simulink model "SF105A_MotCurrRegVltgLimr"  (R2013b)
settings: Solver=FixedStepDiscrete  SolverMode=SingleTasking  StartTime=0.0  StopTime=1  FixedStep=0.00025  RelTol=1e-3
undefined symbols (not defined in the file): ARCHGLBPRM_2OVERSQRT3_ULS_F32, ARCHGLBPRM_2PI_ULS_F32, BRDGVLTGHILIM_VOLT_F32, ELECGLBPRM_PWMPERDNOMX2_SEC_F32, F32TOU16OVR2PI_ULS_F32, MotCurrRegCfgCurrLoopSecOrderTrfFctEna, MotCurrRegCfgMotRVirtDax, MotCurrRegCfgMotRVirtQax, MotCurrRegVltgLimrCurrLoaScarSlewRate, MotCurrRegVltgLimrDaxAntiWdupCoeff, MotCurrRegVltgLimrDualEcuLoaScarSlewRate, MotCurrRegVltgLimrIvtrLoaScarSlewRate, MotCurrRegVltgLimrMotCurrPredEna, MotCurrRegVltgLimrMotCurrPredTi, MotCurrRegVltgLimrMotCurrQaxRefMdfnRplEna, MotCurrRegVltgLimrMotVltgBrdgFilEna, MotCurrRegVltgLimrMotVltgDaxIntglHiLim, MotCurrRegVltgLimrMotVltgDaxIntglLoLim, MotCurrRegVltgLimrMotVltgQaxFfFilEna, MotCurrRegVltgLimrMotVltgQaxIntglHiLim, MotCurrRegVltgLimrMotVltgQaxIntglLoLim, MotCurrRegVltgLimrQaxAntiWdupCoeff, MotCurrRegVltgLimrQaxAntiWdupScagDi, MotRefMdlFbCtrlDi, MotRefMdlIvtrDeadTiBrdgVltgSca, SysSt1, ZERO_VOLT_F32
libraries: NxtrLim x15, Fil x4, simulink x3, NxtrMax x2, NxtrMin x2
(part 4 of 5)

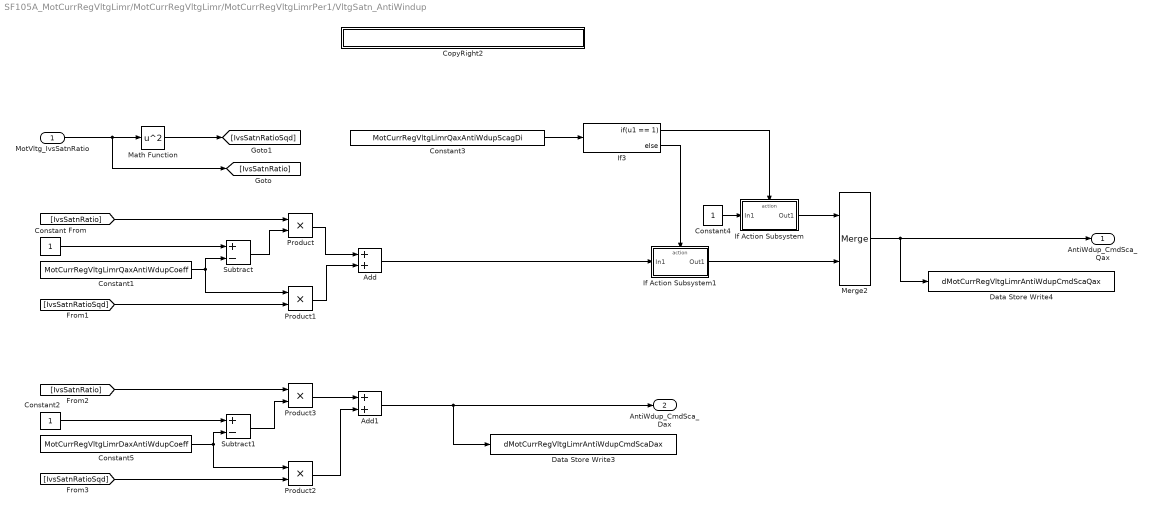
== system SF105A_MotCurrRegVltgLimr/MotCurrRegVltgLimr/MotCurrRegVltgLimrPer1/VltgSatn_AntiWindup ==
  MotVltg_IvsSatnRatio : Inport  RequirementInfo="{'linktype_rmi_doors' '0000bb44 (/E-STEER Core/SubSystem Specifications/Application Functions/SF99/SF105A Current Regulator and Voltage Limiter)' '#SF105A_130' 'true' 'REQ:  SF105A_130' '' ; 'linktype_rmi_doors' '0000bb44 (/E-STEER Core/SubSystem Specifications/Application Functions/SF99/SF105A Current Regulator and Voltage Limiter)' '#SF105A_130' 'true' 'REQ:  SF105A_130' '' } %GIDa_888bca64_0823_4deb_ba1d_307ad11fc636"
  Add : Sum  RequirementInfo="{'linktype_rmi_doors' '0000bb44 (/E-STEER Core/SubSystem Specifications/Application Functions/SF99/SF105A Current Regulator and Voltage Limiter)' '#SF105A_126' 'true' 'REQ:  SF105A_126' '' } %GIDa_812b0983_0c53_4cfa_9a51_643dbc79a070"
  Add1 : Sum  RequirementInfo="{'linktype_rmi_doors' '0000bb44 (/E-STEER Core/SubSystem Specifications/Application Functions/SF99/SF105A Current Regulator and Voltage Limiter)' '#SF105A_130' 'true' 'REQ:  SF105A_130' '' } %GIDa_2674bb96_c0b6_4cdb_b829_01729431041f"
  Constant : Constant  RequirementInfo="{'linktype_rmi_doors' '0000bb44 (/E-STEER Core/SubSystem Specifications/Application Functions/SF99/SF105A Current Regulator and Voltage Limiter)' '#SF105A_126' 'true' 'REQ:  SF105A_126' '' } %GIDa_a4ea031f_79fb_49ac_9d61_2a336d42d170"  OutDataTypeStr=single
  Constant1 : Constant  RequirementInfo="{'linktype_rmi_doors' '0000bb44 (/E-STEER Core/SubSystem Specifications/Application Functions/SF99/SF105A Current Regulator and Voltage Limiter)' '#SF105A_126' 'true' 'REQ:  SF105A_126' '' ; 'linktype_rmi_doors' '0000bb44 (/E-STEER Core/SubSystem Specifications/Application Functions/SF99/SF105A Current Regulator and Voltage Limiter)' '#SF105A_126' 'true' 'REQ:  SF105A_126' '' } %GIDa_f0528501_6455_46bb_9be1_873b38c0945c"  Value=MotCurrRegVltgLimrQaxAntiWdupCoeff
  Constant2 : Constant  RequirementInfo="{'linktype_rmi_doors' '0000bb44 (/E-STEER Core/SubSystem Specifications/Application Functions/SF99/SF105A Current Regulator and Voltage Limiter)' '#SF105A_130' 'true' 'REQ:  SF105A_130' '' } %GIDa_f1e0f24a_4abc_445f_8df3_e7d8a5290d26"  OutDataTypeStr=single
  Constant3 : Constant  RequirementInfo="{'linktype_rmi_doors' '0000bb44 (/E-STEER Core/SubSystem Specifications/Application Functions/SF99/SF105A Current Regulator and Voltage Limiter)' '#SF105A_126' 'true' 'REQ:  SF105A_126' '' } %GIDa_0a590627_be14_4a36_8e32_6ad02ffe62c3"  Value=MotCurrRegVltgLimrQaxAntiWdupScagDi
  Constant4 : Constant  RequirementInfo="{'linktype_rmi_doors' '0000bb44 (/E-STEER Core/SubSystem Specifications/Application Functions/SF99/SF105A Current Regulator and Voltage Limiter)' '#SF105A_126' 'true' 'REQ:  SF105A_126' '' } %GIDa_b2b2de9c_8926_4bf3_ad2c_18100fed640c"  OutDataTypeStr=single
  Constant5 : Constant  RequirementInfo="{'linktype_rmi_doors' '0000bb44 (/E-STEER Core/SubSystem Specifications/Application Functions/SF99/SF105A Current Regulator and Voltage Limiter)' '#SF105A_126' 'true' 'REQ:  SF105A_126' '' ; 'linktype_rmi_doors' '0000bb44 (/E-STEER Core/SubSystem Specifications/Application Functions/SF99/SF105A Current Regulator and Voltage Limiter)' '#SF105A_130' 'true' 'REQ:  SF105A_130' '' } %GIDa_6fe1152d_0e16_4530_a23a_94ed2f7f620d"  Value=MotCurrRegVltgLimrDaxAntiWdupCoeff
  CopyRight2 : Subsystem  Description=|  mask(Copyright Information){none=on}
      | Copyright info block.                                               
      |                                                                     
      | Place copyright information at the top of every subsystem in design.
      mask prompts: none "No parameters"
      mask help: Place copyright information at the top of every subsystem in design.
      mask Display:
      | NxtrConf = 'Nexteer Confidential';
      | 
      | sys = bdroot; %handle for the current model ("system")
      | first = get_param(sys,'Created');
      | if(isempty(first))
      |     first = datestr(now,'yyyy');
      | else
      |     first = first(end-3:end);  %year is last four digits
      | end
      | 
      | last = get_param(sys,'LastModifiedDate');
      | if isempty(last)
      |     last = datestr(now,'yyyy');
      | else
      |     last = last(end-3:end);
      | end
      | 
      | if strcmp(first,last)
      |     fprintf('%s -- Copyright %s Nexteer',NxtrConf,first)
      | else
      |     fprintf('%s -- %s%s- %s Nexteer',NxtrConf,char(169),first,last)
      | end
  Data Store Write3 : DataStoreWrite  RequirementInfo="{'linktype_rmi_doors' '0000bb44 (/E-STEER Core/SubSystem Specifications/Application Functions/SF99/SF105A Current Regulator and Voltage Limiter)' '#SF105A_141' 'true' 'REQ:  SF105A_141' '' } %GIDa_d69d978d_8d8c_4eb5_8eb7_5cf010971c8b"  DataStoreName=dMotCurrRegVltgLimrAntiWdupCmdScaDax
  Data Store Write4 : DataStoreWrite  RequirementInfo="{'linktype_rmi_doors' '0000bb44 (/E-STEER Core/SubSystem Specifications/Application Functions/SF99/SF105A Current Regulator and Voltage Limiter)' '#SF105A_141' 'true' 'REQ:  SF105A_141' '' } %GIDa_9849020c_0cb1_40e6_a462_20415501e4e7"  DataStoreName=dMotCurrRegVltgLimrAntiWdupCmdScaQax
  If Action Subsystem : Subsystem  RequirementInfo="{'linktype_rmi_doors' '0000bb44 (/E-STEER Core/SubSystem Specifications/Application Functions/SF99/SF105A Current Regulator and Voltage Limiter)' '#SF105A_126' 'true' 'REQ:  SF105A_126' '' } %GIDa_c49f3131_c39a_4483_bd39_15998722cd10"  TreatAsAtomicUnit=on
  If Action Subsystem1 : Subsystem  RequirementInfo="{'linktype_rmi_doors' '0000bb44 (/E-STEER Core/SubSystem Specifications/Application Functions/SF99/SF105A Current Regulator and Voltage Limiter)' '#SF105A_126' 'true' 'REQ:  SF105A_126' '' } %GIDa_0be6e736_8039_4cb8_9da1_1d96e36153a9"  TreatAsAtomicUnit=on
  If3 : If  RequirementInfo="{'linktype_rmi_doors' '0000bb44 (/E-STEER Core/SubSystem Specifications/Application Functions/SF99/SF105A Current Regulator and Voltage Limiter)' '#SF105A_126' 'true' 'REQ:  SF105A_126' '' } %GIDa_dbf56d85_10ab_48c7_a6a3_82cb7cfa18de"  IfExpression=u1 == 1
  Math Function : Math  RequirementInfo="{'linktype_rmi_doors' '0000bb44 (/E-STEER Core/SubSystem Specifications/Application Functions/SF99/SF105A Current Regulator and Voltage Limiter)' '#SF105A_130' 'true' 'REQ:  SF105A_130' '' ; 'linktype_rmi_doors' '0000bb44 (/E-STEER Core/SubSystem Specifications/Application Functions/SF99/SF105A Current Regulator and Voltage Limiter)' '#SF105A_130' 'true' 'REQ:  SF105A_130' '' } %GIDa_b09f1dfa_1331_43ca_8f8b_9feb85653759"  Operator=square  SaturateOnIntegerOverflow=on
  Merge2 : Merge  RequirementInfo="{'linktype_rmi_doors' '0000bb44 (/E-STEER Core/SubSystem Specifications/Application Functions/SF99/SF105A Current Regulator and Voltage Limiter)' '#SF105A_126' 'true' 'REQ:  SF105A_126' '' } %GIDa_8d5f9f4e_85d5_4273_905f_4ef98e59c94a"
  Product : Product  RequirementInfo="{'linktype_rmi_doors' '0000bb44 (/E-STEER Core/SubSystem Specifications/Application Functions/SF99/SF105A Current Regulator and Voltage Limiter)' '#SF105A_126' 'true' 'REQ:  SF105A_126' '' } %GIDa_ea6027c8_8a1b_4f13_be09_e5e1cad10d1f"
  Product1 : Product  RequirementInfo="{'linktype_rmi_doors' '0000bb44 (/E-STEER Core/SubSystem Specifications/Application Functions/SF99/SF105A Current Regulator and Voltage Limiter)' '#SF105A_126' 'true' 'REQ:  SF105A_126' '' } %GIDa_f8ee43f2_9342_474e_acda_6fc019895fb8"
  Product2 : Product  RequirementInfo="{'linktype_rmi_doors' '0000bb44 (/E-STEER Core/SubSystem Specifications/Application Functions/SF99/SF105A Current Regulator and Voltage Limiter)' '#SF105A_130' 'true' 'REQ:  SF105A_130' '' } %GIDa_1c2ad4c0_5990_4d45_bbe5_57d9582fe383"
  Product3 : Product  RequirementInfo="{'linktype_rmi_doors' '0000bb44 (/E-STEER Core/SubSystem Specifications/Application Functions/SF99/SF105A Current Regulator and Voltage Limiter)' '#SF105A_130' 'true' 'REQ:  SF105A_130' '' } %GIDa_0fc5ec00_cbe3_4725_98f5_b8cec8d7b237"
  Subtract : Sum  RequirementInfo="{'linktype_rmi_doors' '0000bb44 (/E-STEER Core/SubSystem Specifications/Application Functions/SF99/SF105A Current Regulator and Voltage Limiter)' '#SF105A_126' 'true' 'REQ:  SF105A_126' '' } %GIDa_ed1d9f08_fe01_45f1_add5_02a80c037d9d"  Inputs=+-
  Subtract1 : Sum  RequirementInfo="{'linktype_rmi_doors' '0000bb44 (/E-STEER Core/SubSystem Specifications/Application Functions/SF99/SF105A Current Regulator and Voltage Limiter)' '#SF105A_130' 'true' 'REQ:  SF105A_130' '' } %GIDa_badc02ff_cfe5_4c0b_9d95_39b5b5fe7a5f"  Inputs=+-
  AntiWdup_CmdSca_Qax : Outport  RequirementInfo="{'linktype_rmi_doors' '0000bb44 (/E-STEER Core/SubSystem Specifications/Application Functions/SF99/SF105A Current Regulator and Voltage Limiter)' '#SF105A_126' 'true' 'REQ:  SF105A_126' '' } %GIDa_d17ed289_17c6_4f50_a1dc_ba7a5b94eaaa"
  AntiWdup_CmdSca_Dax : Outport  RequirementInfo="{'linktype_rmi_doors' '0000bb44 (/E-STEER Core/SubSystem Specifications/Application Functions/SF99/SF105A Current Regulator and Voltage Limiter)' '#SF105A_130' 'true' 'REQ:  SF105A_130' '' } %GIDa_6b63b34d_3c6d_43f2_8b57_6061e5110967"  Port=2
  wires:
  [IvsSatnRatioSqd] -> Product2/2
  [IvsSatnRatio] -> Product3/1
  [IvsSatnRatio] -> Product/1
  [IvsSatnRatioSqd] -> Product1/2
  Math Function/1 -> [IvsSatnRatioSqd]
  Product2/1 -> Add1/2
  Product3/1 -> Add1/1
  Subtract1/1 -> Product3/2
  MotVltg_IvsSatnRatio/1 -> Math Function/1, [IvsSatnRatio]
  Constant5/1 -> Subtract1/2, Product2/1
  Constant2/1 -> Subtract1/1
  Product1/1 -> Add/2
  Product/1 -> Add/1
  Subtract/1 -> Product/2
  Constant1/1 -> Product1/1, Subtract/2
  Constant/1 -> Subtract/1
  Merge2/1 -> AntiWdup_CmdSca_Qax/1, Data Store Write4/1
  If Action Subsystem1/1(Out1) -> Merge2/2
  If Action Subsystem/1(Out1) -> Merge2/1
  If3/2 -> If Action Subsystem1/Action
  If3/1 -> If Action Subsystem/Action
  Constant4/1 -> If Action Subsystem/1(In1)
  Add/1 -> If Action Subsystem1/1(In1)
  Constant3/1 -> If3/1
  Add1/1 -> AntiWdup_CmdSca_Dax/1, Data Store Write3/1

== system SF105A_MotCurrRegVltgLimr/MotCurrRegVltgLimr/MotCurrRegVltgLimrPer1/Calc_Limit_Cmd_Final/BrdgVltgFiltering ==
  note: The Ic of MotVltgBrdgLpFil PIM in MotCurrRegVltgLimrInit1 takes care of
      | the filter output init requirement.
  note: The initial value of the filter output should be BRDGVLTDFT_VOLT_F32,
      | in addition to setting the initial value of the state variable as specified.
  BrdgVltg : Inport  RequirementInfo="{'linktype_rmi_doors' '0000bb44 (/E-STEER Core/SubSystem Specifications/Application Functions/SF99/SF105A Current Regulator and Voltage Limiter)' '#SF105A_135' 'true' 'REQ:  SF105A_135' '' } %GIDa_864daba2_2840_4178_946c_2ce536d951a0"
  CopyRight1 : Subsystem  Description=|  mask(Copyright Information){none=on}
      | Copyright info block.                                               
      |                                                                     
      | Place copyright information at the top of every subsystem in design.
      mask prompts: none "No parameters"
      mask help: Place copyright information at the top of every subsystem in design.
      mask Display:
      | NxtrConf = 'Nexteer Confidential';
      | 
      | sys = bdroot; %handle for the current model ("system")
      | first = get_param(sys,'Created');
      | if(isempty(first))
      |     first = datestr(now,'yyyy');
      | else
      |     first = first(end-3:end);  %year is last four digits
      | end
      | 
      | last = get_param(sys,'LastModifiedDate');
      | if isempty(last)
      |     last = datestr(now,'yyyy');
      | else
      |     last = last(end-3:end);
      | end
      | 
      | if strcmp(first,last)
      |     fprintf('%s -- Copyright %s Nexteer',NxtrConf,first)
      | else
      |     fprintf('%s -- %s%s- %s Nexteer',NxtrConf,char(169),first,last)
      | end
  Data Store Write : DataStoreWrite  DataStoreName=dMotCurrRegVltgLimrMotVltgBrdgFild
  FilLpUpdOutp : Fil/FilLpUpdOutp  RequirementInfo="{'linktype_rmi_doors' '0000bb44 (/E-STEER Core/SubSystem Specifications/Application Functions/SF99/SF105A Current Regulator and Voltage Limiter)' '#SF105A_187' 'true' 'REQ:  SF105A_187' '' } %GIDa_46ddaace_b65f_4907_a29c_a4e4204d39a8"  StVar=MotVltgBrdgLpFil
      settings: AttributesFormatString=StVar: %<StVar>
  If : If  RequirementInfo="{'linktype_rmi_doors' '0000bb44 (/E-STEER Core/SubSystem Specifications/Application Functions/SF99/SF105A Current Regulator and Voltage Limiter)' '#SF105A_187' 'true' 'REQ:  SF105A_187' '' } %GIDa_b268bc1a_d9d5_470b_b0ef_ff6c9bd052c7"  IfExpression=u1
  If Action Subsystem : Subsystem  RequirementInfo="{'linktype_rmi_doors' '0000bb44 (/E-STEER Core/SubSystem Specifications/Application Functions/SF99/SF105A Current Regulator and Voltage Limiter)' '#SF105A_187' 'true' 'REQ:  SF105A_187' '' } %GIDa_971e247e_23b6_4861_af8f_f82189af1b5d"  TreatAsAtomicUnit=on
  If Action Subsystem1 : Subsystem  RequirementInfo="{'linktype_rmi_doors' '0000bb44 (/E-STEER Core/SubSystem Specifications/Application Functions/SF99/SF105A Current Regulator and Voltage Limiter)' '#SF105A_187' 'true' 'REQ:  SF105A_187' '' } %GIDa_df7b0156_11d7_47ef_b6b6_7cc2d22d8aaa"  TreatAsAtomicUnit=on
  LimStat_f32 : NxtrLim/LimStat_f32  RequirementInfo="{'linktype_rmi_doors' '0000bb44 (/E-STEER Core/SubSystem Specifications/Application Functions/SF99/SF105A Current Regulator and Voltage Limiter)' '#SF105A_196' 'true' 'REQ:  SF105A_196' '' } %GIDa_867aa617_d9e8_4ea6_beda_d730be2610d8"  LoLim=BRDGVLTGLOLIM_VOLT_F32  HiLim=BRDGVLTGHILIM_VOLT_F32
      settings: AttributesFormatString=|
      | Low Limit: %<LoLim>
      | High Limit:%<HiLim>
  Merge : Merge  RequirementInfo="{'linktype_rmi_doors' '0000bb44 (/E-STEER Core/SubSystem Specifications/Application Functions/SF99/SF105A Current Regulator and Voltage Limiter)' '#SF105A_187' 'true' 'REQ:  SF105A_187' '' } %GIDa_7831497a_f68e_4bbe_8502_8e5fd0963902"
  k_MtrVel_Offset1 : Constant  RequirementInfo="{'linktype_rmi_doors' '0000bb44 (/E-STEER Core/SubSystem Specifications/Application Functions/SF99/SF105A Current Regulator and Voltage Limiter)' '#SF105A_115' 'true' 'REQ:  SF105A_115' '' } %GIDa_cb62c815_145d_482f_a77a_dcb58bda804e"  Value=MotCurrRegVltgLimrMotVltgBrdgFilEna
  BrdgVltgFild : Outport  RequirementInfo="{'linktype_rmi_doors' '0000bb44 (/E-STEER Core/SubSystem Specifications/Application Functions/SF99/SF105A Current Regulator and Voltage Limiter)' '#SF105A_73' 'true' 'REQ:  SF105A_73' '' } %GIDa_48ce5847_960a_4607_a314_b555c1a99ed4"
  wires:
  BrdgVltg/1 -> If Action Subsystem1/1(In1), FilLpUpdOutp/1
  FilLpUpdOutp/1 -> LimStat_f32/1
  k_MtrVel_Offset1/1 -> If/1
  LimStat_f32/1 -> If Action Subsystem/1(In1)
  If/1 -> If Action Subsystem/Action
  If/2 -> If Action Subsystem1/Action
  If Action Subsystem/1(Out1) -> Merge/1
  If Action Subsystem1/1(Out1) -> Merge/2
  Merge/1 -> Data Store Write/1, BrdgVltgFild/1

== system SF105A_MotCurrRegVltgLimr/MotCurrRegVltgLimr/MotCurrRegVltgLimrPer1/Calc_Limit_Cmd_Final/CopyRight2 ==

== system SF105A_MotCurrRegVltgLimr/MotCurrRegVltgLimr/MotCurrRegVltgLimrPer1/Calc_Limit_Cmd_Final/PhaAdvCalc ==
  note: We need a U0P16 datatype and it is acheived by using
      | 'F32TOU16OVR2PI_ULS_F32' constant multiplication.
      |
      | So we just need to convert a float value to fixed point value.
  MotVltg_PreLim_Dax : Inport  RequirementInfo="{'linktype_rmi_doors' '0000bb44 (/E-STEER Core/SubSystem Specifications/Application Functions/SF99/SF105A Current Regulator and Voltage Limiter)' '#SF105A_121' 'true' 'REQ:  SF105A_121' '' } %GIDa_bdcfd20c_9724_4f7f_8f44_b138d6ea85d6"
  InMotVltg_PreLim_Qax : Inport  RequirementInfo="{'linktype_rmi_doors' '0000bb44 (/E-STEER Core/SubSystem Specifications/Application Functions/SF99/SF105A Current Regulator and Voltage Limiter)' '#SF105A_121' 'true' 'REQ:  SF105A_121' '' } %GIDa_24b87ca2_4d87_4994_b5fa_a1b91e2e207b"  Port=2
  MotAgElecDly : Inport  RequirementInfo="{'linktype_rmi_doors' '0000bb44 (/E-STEER Core/SubSystem Specifications/Application Functions/SF99/SF105A Current Regulator and Voltage Limiter)' '#SF105A_121' 'true' 'REQ:  SF105A_121' '' } %GIDa_d623a715_ec5b_4f45_bad7_6c2e1720bc37"  Port=3
  Add 2 Pi : Subsystem  RequirementInfo="{'linktype_rmi_doors' '0000bb44 (/E-STEER Core/SubSystem Specifications/Application Functions/SF99/SF105A Current Regulator and Voltage Limiter)' '#SF105A_122' 'true' 'REQ:  SF105A_122' '' } %GIDa_bec4bd50_a64b_49aa_a5f2_b456e732021b"  TreatAsAtomicUnit=on
  Add3 : Sum  RequirementInfo="{'linktype_rmi_doors' '0000bb44 (/E-STEER Core/SubSystem Specifications/Application Functions/SF99/SF105A Current Regulator and Voltage Limiter)' '#SF105A_121' 'true' 'REQ:  SF105A_121' '' ; 'linktype_rmi_doors' '0000bb44 (/E-STEER Core/SubSystem Specifications/Application Functions/SF99/SF105A Current Regulator and Voltage Limiter)' '#SF105A_121' 'true' 'REQ:  SF105A_121' '' } %GIDa_c56e8bdb_47aa_4567_8a35_dd84849c0b34"
  Constant : Constant  RequirementInfo="{'linktype_rmi_doors' '0000bb44 (/E-STEER Core/SubSystem Specifications/Application Functions/SF99/SF105A Current Regulator and Voltage Limiter)' '#SF105A_122' 'true' 'REQ:  SF105A_122' '' } %GIDa_d713a677_ab63_42ce_9fe8_5d59c338472e"  Value=ARCHGLBPRM_2PI_ULS_F32
  Constant1 : Constant  RequirementInfo="{'linktype_rmi_doors' '0000bb44 (/E-STEER Core/SubSystem Specifications/Application Functions/SF99/SF105A Current Regulator and Voltage Limiter)' '#SF105A_175' 'true' 'REQ:  SF105A_175' '' } %GIDa_008443f9_f6f6_4afb_be91_a11b98c8e251"  Value=F32TOU16OVR2PI_ULS_F32
  Constant2 : Constant  RequirementInfo="{'linktype_rmi_doors' '0000bb44 (/E-STEER Core/SubSystem Specifications/Application Functions/SF99/SF105A Current Regulator and Voltage Limiter)' '#SF105A_122' 'true' 'REQ:  SF105A_122' '' } %GIDa_8b075e1e_a827_4df9_9ee2_e9524eb3af15"  Value=0
  CopyRight2 : Subsystem  Description=|  mask(Copyright Information){none=on}
      | Copyright info block.                                               
      |                                                                     
      | Place copyright information at the top of every subsystem in design.
      mask prompts: none "No parameters"
      mask help: Place copyright information at the top of every subsystem in design.
      mask Display:
      | NxtrConf = 'Nexteer Confidential';
      | 
      | sys = bdroot; %handle for the current model ("system")
      | first = get_param(sys,'Created');
      | if(isempty(first))
      |     first = datestr(now,'yyyy');
      | else
      |     first = first(end-3:end);  %year is last four digits
      | end
      | 
      | last = get_param(sys,'LastModifiedDate');
      | if isempty(last)
      |     last = datestr(now,'yyyy');
      | else
      |     last = last(end-3:end);
      | end
      | 
      | if strcmp(first,last)
      |     fprintf('%s -- Copyright %s Nexteer',NxtrConf,first)
      | else
      |     fprintf('%s -- %s%s- %s Nexteer',NxtrConf,char(169),first,last)
      | end
  Data Store Write2 : DataStoreWrite  DataStoreName=dMotCurrRegVltgLimrPhaAdvPreDly
  Data Type Conversion : DataTypeConversion  OutDataTypeStr=uint16
  Do Nothing : Subsystem  RequirementInfo="{'linktype_rmi_doors' '0000bb44 (/E-STEER Core/SubSystem Specifications/Application Functions/SF99/SF105A Current Regulator and Voltage Limiter)' '#SF105A_122' 'true' 'REQ:  SF105A_122' '' } %GIDa_39de0701_934e_4724_8bf7_c6902dec6381"  TreatAsAtomicUnit=on
  If : If  RequirementInfo="{'linktype_rmi_doors' '0000bb44 (/E-STEER Core/SubSystem Specifications/Application Functions/SF99/SF105A Current Regulator and Voltage Limiter)' '#SF105A_122' 'true' 'REQ:  SF105A_122' '' } %GIDa_6debbc16_2f73_4bff_b693_245b5406855e"  NumInputs=2  IfExpression=u1 == 1  ElseIfExpressions=u2 == 1
  LimStat_f32 : NxtrLim/LimStat_f32  LoLim=PHAADVLOLIM_MOTREV_F32  HiLim=PHAADVHILIM_MOTREV_F32
      settings: AttributesFormatString=|
      | Low Limit: %<LoLim>
      | High Limit:%<HiLim>
  Merge : Merge  RequirementInfo="{'linktype_rmi_doors' '0000bb44 (/E-STEER Core/SubSystem Specifications/Application Functions/SF99/SF105A Current Regulator and Voltage Limiter)' '#SF105A_122' 'true' 'REQ:  SF105A_122' '' } %GIDa_6557e4a1_f45b_486a_b2f8_481b6d465a1f"  Inputs=3
  Product : Product  RequirementInfo="{'linktype_rmi_doors' '0000bb44 (/E-STEER Core/SubSystem Specifications/Application Functions/SF99/SF105A Current Regulator and Voltage Limiter)' '#SF105A_175' 'true' 'REQ:  SF105A_175' '' } %GIDa_bd389a6c_476a_46fc_af98_4788a351a6be"
  Relational Operator : RelationalOperator  RequirementInfo="{'linktype_rmi_doors' '0000bb44 (/E-STEER Core/SubSystem Specifications/Application Functions/SF99/SF105A Current Regulator and Voltage Limiter)' '#SF105A_122' 'true' 'REQ:  SF105A_122' '' } %GIDa_28fbb344_18a1_4c6b_a257_0afea322ddf0"  OutDataTypeStr=boolean
  Relational Operator1 : RelationalOperator  RequirementInfo="{'linktype_rmi_doors' '0000bb44 (/E-STEER Core/SubSystem Specifications/Application Functions/SF99/SF105A Current Regulator and Voltage Limiter)' '#SF105A_122' 'true' 'REQ:  SF105A_122' '' } %GIDa_85166377_0294_4ce9_b13e_1ed5624f31e0"  Operator=<  OutDataTypeStr=boolean
  Subtract 2 Pi : Subsystem  RequirementInfo="{'linktype_rmi_doors' '0000bb44 (/E-STEER Core/SubSystem Specifications/Application Functions/SF99/SF105A Current Regulator and Voltage Limiter)' '#SF105A_122' 'true' 'REQ:  SF105A_122' '' } %GIDa_cb336f9e_1bd0_4f20_8c52_7fd85ab16bd3"  TreatAsAtomicUnit=on
  atan2 : Trigonometry  RequirementInfo="{'linktype_rmi_doors' '0000bb44 (/E-STEER Core/SubSystem Specifications/Application Functions/SF99/SF105A Current Regulator and Voltage Limiter)' '#SF105A_121' 'true' 'REQ:  SF105A_121' '' } %GIDa_4538e4d2_8506_4d02_a08e_4739cbb91fa4"  Operator=atan2
  PhaAdv : Outport  RequirementInfo="{'linktype_rmi_doors' '0000bb44 (/E-STEER Core/SubSystem Specifications/Application Functions/SF99/SF105A Current Regulator and Voltage Limiter)' '#SF105A_175' 'true' 'REQ:  SF105A_175' '' } %GIDa_681c00ed_fb07_4e1f_a6af_37fdf2821b8b"
  wires:
  InMotVltg_PreLim_Qax/1 -> atan2/2
  MotVltg_PreLim_Dax/1 -> atan2/1
  atan2/1 -> Add3/1
  MotAgElecDly/1 -> Add3/2
  Constant1/1 -> Product/2
  Add3/1 -> [PhaAdvPreDly], Relational Operator1/1, Relational Operator/1
  Product/1 -> LimStat_f32/1
  Data Type Conversion/1 -> PhaAdv/1
  Constant/1 -> Relational Operator/2
  Relational Operator/1 -> If/1
  Constant2/1 -> Relational Operator1/2
  Relational Operator1/1 -> If/2
  If/1 -> Subtract 2 Pi/Action
  If/2 -> Add 2 Pi/Action
  If/3 -> Do Nothing/Action
  [PhaAdvPreDly] -> Do Nothing/1(In1)
  [PhaAdvPreDly] -> Add 2 Pi/1(In1)
  [PhaAdvPreDly] -> Subtract 2 Pi/1(In1)
  Add 2 Pi/1(Out1) -> Merge/2
  Subtract 2 Pi/1(Out1) -> Merge/1
  Do Nothing/1(Out1) -> Merge/3
  Merge/1 -> Product/1, Data Store Write2/1
  LimStat_f32/1 -> Data Type Conversion/1

== system SF105A_MotCurrRegVltgLimr/MotCurrRegVltgLimr/MotCurrRegVltgLimrPer1/Calc_Limit_Cmd_Final/VltgCalcFinal ==
  VltgSatnIvsRatio : Inport  RequirementInfo="{'linktype_rmi_doors' '0000bb44 (/E-STEER Core/SubSystem Specifications/Application Functions/SF99/SF105A Current Regulator and Voltage Limiter)' '#SF105A_118' 'true' 'REQ:  SF105A_118' '' } %GIDa_92808367_e524_470e_8cbd_a129a7d2d4b3"
  MotVltg_CmdPreLim : Inport  RequirementInfo="{'linktype_rmi_doors' '0000bb44 (/E-STEER Core/SubSystem Specifications/Application Functions/SF99/SF105A Current Regulator and Voltage Limiter)' '#SF105A_118' 'true' 'REQ:  SF105A_118' '' } %GIDa_a07a3682_c8d9_4fb3_b50c_c57fed612463"  Port=2
  MotVltg_PreLim_Qax : Inport  RequirementInfo="{'linktype_rmi_doors' '0000bb44 (/E-STEER Core/SubSystem Specifications/Application Functions/SF99/SF105A Current Regulator and Voltage Limiter)' '#SF105A_118' 'true' 'REQ:  SF105A_118' '' } %GIDa_dd71d561_8f03_4624_bfe4_a63edcd030a2"  Port=3
  MotVltg_PreLim_Dax : Inport  RequirementInfo="{'linktype_rmi_doors' '0000bb44 (/E-STEER Core/SubSystem Specifications/Application Functions/SF99/SF105A Current Regulator and Voltage Limiter)' '#SF105A_118' 'true' 'REQ:  SF105A_118' '' } %GIDa_28090249_119c_4353_905a_27cfc52c482c"  Port=4
  CopyRight2 : Subsystem  Description=|  mask(Copyright Information){none=on}
      | Copyright info block.                                               
      |                                                                     
      | Place copyright information at the top of every subsystem in design.
      mask prompts: none "No parameters"
      mask help: Place copyright information at the top of every subsystem in design.
      mask Display:
      | NxtrConf = 'Nexteer Confidential';
      | 
      | sys = bdroot; %handle for the current model ("system")
      | first = get_param(sys,'Created');
      | if(isempty(first))
      |     first = datestr(now,'yyyy');
      | else
      |     first = first(end-3:end);  %year is last four digits
      | end
      | 
      | last = get_param(sys,'LastModifiedDate');
      | if isempty(last)
      |     last = datestr(now,'yyyy');
      | else
      |     last = last(end-3:end);
      | end
      | 
      | if strcmp(first,last)
      |     fprintf('%s -- Copyright %s Nexteer',NxtrConf,first)
      | else
      |     fprintf('%s -- %s%s- %s Nexteer',NxtrConf,char(169),first,last)
      | end
  Product : Product  RequirementInfo="{'linktype_rmi_doors' '0000bb44 (/E-STEER Core/SubSystem Specifications/Application Functions/SF99/SF105A Current Regulator and Voltage Limiter)' '#SF105A_118' 'true' 'REQ:  SF105A_118' '' } %GIDa_26ce41e9_a68c_40ea_8d80_c25ab29a05d8"
  Product1 : Product  RequirementInfo="{'linktype_rmi_doors' '0000bb44 (/E-STEER Core/SubSystem Specifications/Application Functions/SF99/SF105A Current Regulator and Voltage Limiter)' '#SF105A_118' 'true' 'REQ:  SF105A_118' '' } %GIDa_03fdffe1_9228_4be0_96dd_0c0f485f5b41"
  Product2 : Product  RequirementInfo="{'linktype_rmi_doors' '0000bb44 (/E-STEER Core/SubSystem Specifications/Application Functions/SF99/SF105A Current Regulator and Voltage Limiter)' '#SF105A_118' 'true' 'REQ:  SF105A_118' '' } %GIDa_71405c77_fbaf_47db_89a9_468137e99d7f"
  MotVltg_Qax : Outport  RequirementInfo="{'linktype_rmi_doors' '0000bb44 (/E-STEER Core/SubSystem Specifications/Application Functions/SF99/SF105A Current Regulator and Voltage Limiter)' '#SF105A_118' 'true' 'REQ:  SF105A_118' '' } %GIDa_497cbdd0_9069_488d_a909_6a66b2256717"
  MotVltg_Dax : Outport  RequirementInfo="{'linktype_rmi_doors' '0000bb44 (/E-STEER Core/SubSystem Specifications/Application Functions/SF99/SF105A Current Regulator and Voltage Limiter)' '#SF105A_118' 'true' 'REQ:  SF105A_118' '' } %GIDa_d46a1546_21ba_4d6d_bf0a_a4d6c3cb79f7"  Port=2
  MotVltg_Cmd : Outport  RequirementInfo="{'linktype_rmi_doors' '0000bb44 (/E-STEER Core/SubSystem Specifications/Application Functions/SF99/SF105A Current Regulator and Voltage Limiter)' '#SF105A_118' 'true' 'REQ:  SF105A_118' '' } %GIDa_063fcbc4_0213_4015_8c39_ad9bdc608897"  Port=3
  wires:
  VltgSatnIvsRatio/1 -> Product2/1, Product1/1, Product/1
  MotVltg_PreLim_Qax/1 -> Product/2
  MotVltg_PreLim_Dax/1 -> Product1/2
  MotVltg_CmdPreLim/1 -> Product2/2
  Product2/1 -> MotVltg_Cmd/1
  Product/1 -> MotVltg_Qax/1
  Product1/1 -> MotVltg_Dax/1

== system SF105A_MotCurrRegVltgLimr/MotCurrRegVltgLimr/MotCurrRegVltgLimrPer1/Calc_Limit_Cmd_Final/VltgSatnIvsRatioCalc ==
  MotVltg_CmdPreLim : Inport  RequirementInfo="{'linktype_rmi_doors' '0000bb44 (/E-STEER Core/SubSystem Specifications/Application Functions/SF99/SF105A Current Regulator and Voltage Limiter)' '#SF105A_172' 'true' 'REQ:  SF105A_172' '' } %GIDa_684f735c_8aea_44ce_8e78_2ff6c7d19092"
  BrdgVltgScad : Inport  RequirementInfo="{'linktype_rmi_doors' '0000bb44 (/E-STEER Core/SubSystem Specifications/Application Functions/SF99/SF105A Current Regulator and Voltage Limiter)' '#SF105A_172' 'true' 'REQ:  SF105A_172' '' } %GIDa_4bf051e1_6c4d_42ea_b111_163ebfa9da75"  Port=2
  CalculateInverse : Subsystem  RequirementInfo="{'linktype_rmi_doors' '0000bb44 (/E-STEER Core/SubSystem Specifications/Application Functions/SF99/SF105A Current Regulator and Voltage Limiter)' '#SF105A_172' 'true' 'REQ:  SF105A_172' '' } %GIDa_d0de5c6b_735e_4ecd_891d_ea6812644bae"  TreatAsAtomicUnit=on
  Constant : Constant  RequirementInfo="{'linktype_rmi_doors' '0000bb44 (/E-STEER Core/SubSystem Specifications/Application Functions/SF99/SF105A Current Regulator and Voltage Limiter)' '#SF105A_172' 'true' 'REQ:  SF105A_172' '' } %GIDa_edd7435b_cecd_4143_9c35_7736d110d5d6"  OutDataTypeStr=single
  Constant1 : Constant  RequirementInfo="{'linktype_rmi_doors' '0000bb44 (/E-STEER Core/SubSystem Specifications/Application Functions/SF99/SF105A Current Regulator and Voltage Limiter)' '#SF105A_172' 'true' 'REQ:  SF105A_172' '' } %GIDa_c7a7d9b4_4354_4293_816c_f1c957552244"  SampleTime=-1
  CopyRight2 : Subsystem  Description=|  mask(Copyright Information){none=on}
      | Copyright info block.                                               
      |                                                                     
      | Place copyright information at the top of every subsystem in design.
      mask prompts: none "No parameters"
      mask help: Place copyright information at the top of every subsystem in design.
      mask Display:
      | NxtrConf = 'Nexteer Confidential';
      | 
      | sys = bdroot; %handle for the current model ("system")
      | first = get_param(sys,'Created');
      | if(isempty(first))
      |     first = datestr(now,'yyyy');
      | else
      |     first = first(end-3:end);  %year is last four digits
      | end
      | 
      | last = get_param(sys,'LastModifiedDate');
      | if isempty(last)
      |     last = datestr(now,'yyyy');
      | else
      |     last = last(end-3:end);
      | end
      | 
      | if strcmp(first,last)
      |     fprintf('%s -- Copyright %s Nexteer',NxtrConf,first)
      | else
      |     fprintf('%s -- %s%s- %s Nexteer',NxtrConf,char(169),first,last)
      | end
  Data Store Write : DataStoreWrite  RequirementInfo="{'linktype_rmi_doors' '0000bb44 (/E-STEER Core/SubSystem Specifications/Application Functions/SF99/SF105A Current Regulator and Voltage Limiter)' '#SF105A_172' 'true' 'REQ:  SF105A_172' '' } %GIDa_840b44d0_598e_446e_ad7f_c7f747c6936b"  DataStoreName=dMotCurrRegVltgLimrMotVltgSatnRat
  Data Store Write2 : DataStoreWrite  RequirementInfo="{'linktype_rmi_doors' '0000bb44 (/E-STEER Core/SubSystem Specifications/Application Functions/SF99/SF105A Current Regulator and Voltage Limiter)' '#SF105A_172' 'true' 'REQ:  SF105A_172' '' } %GIDa_ed39e316_c5b6_4481_974f_e9ae5580d632"  DataStoreName=dMotCurrRegVltgLimrMotVltgSatnIvsRat
  Divide : Product  RequirementInfo="{'linktype_rmi_doors' '0000bb44 (/E-STEER Core/SubSystem Specifications/Application Functions/SF99/SF105A Current Regulator and Voltage Limiter)' '#SF105A_172' 'true' 'REQ:  SF105A_172' '' } %GIDa_44f32095_3d9d_4499_98ae_2bd00f6cceed"  Inputs=*/
  If Action Subsystem1 : Subsystem  RequirementInfo="{'linktype_rmi_doors' '0000bb44 (/E-STEER Core/SubSystem Specifications/Application Functions/SF99/SF105A Current Regulator and Voltage Limiter)' '#SF105A_172' 'true' 'REQ:  SF105A_172' '' } %GIDa_6b5305bd_9183_407b_9534_f292048cbacc"  TreatAsAtomicUnit=on
  If1 : If  RequirementInfo="{'linktype_rmi_doors' '0000bb44 (/E-STEER Core/SubSystem Specifications/Application Functions/SF99/SF105A Current Regulator and Voltage Limiter)' '#SF105A_172' 'true' 'REQ:  SF105A_172' '' } %GIDa_751ed6f9_9f55_4a86_a629_19bbb6ba7dee"  IfExpression=u1 == 1
  Merge : Merge  RequirementInfo="{'linktype_rmi_doors' '0000bb44 (/E-STEER Core/SubSystem Specifications/Application Functions/SF99/SF105A Current Regulator and Voltage Limiter)' '#SF105A_172' 'true' 'REQ:  SF105A_172' '' } %GIDa_2edd8899_22ef_4ae8_a025_f7c7bcc183b0"
  Relational Operator : RelationalOperator  RequirementInfo="{'linktype_rmi_doors' '0000bb44 (/E-STEER Core/SubSystem Specifications/Application Functions/SF99/SF105A Current Regulator and Voltage Limiter)' '#SF105A_172' 'true' 'REQ:  SF105A_172' '' } %GIDa_87e83870_50f1_4566_857e_e61d6254e9f1"  Operator=>  OutDataTypeStr=boolean
  VltgSatnIvsRatio : Outport  RequirementInfo="{'linktype_rmi_doors' '0000bb44 (/E-STEER Core/SubSystem Specifications/Application Functions/SF99/SF105A Current Regulator and Voltage Limiter)' '#SF105A_172' 'true' 'REQ:  SF105A_172' '' } %GIDa_c62c300b_7cef_4326_956b_1370e7f7734a"
  wires:
  MotVltg_CmdPreLim/1 -> Divide/1
  Constant1/1 -> Relational Operator/2
  Relational Operator/1 -> If1/1
  If1/1 -> CalculateInverse/Action
  If1/2 -> If Action Subsystem1/Action
  Constant/1 -> If Action Subsystem1/1(In1)
  Merge/1 -> Data Store Write2/1, VltgSatnIvsRatio/1
  CalculateInverse/1(VltgSatnIvsRatio) -> Merge/1
  If Action Subsystem1/1(Out1) -> Merge/2
  BrdgVltgScad/1 -> Divide/2
  Divide/1 -> CalculateInverse/1(VltgSatnRatio), Data Store Write/1, Relational Operator/1

== system SF105A_MotCurrRegVltgLimr/MotCurrRegVltgLimr/MotCurrRegVltgLimrPer1/Dax_Vltg_Sum/CopyRight2 ==

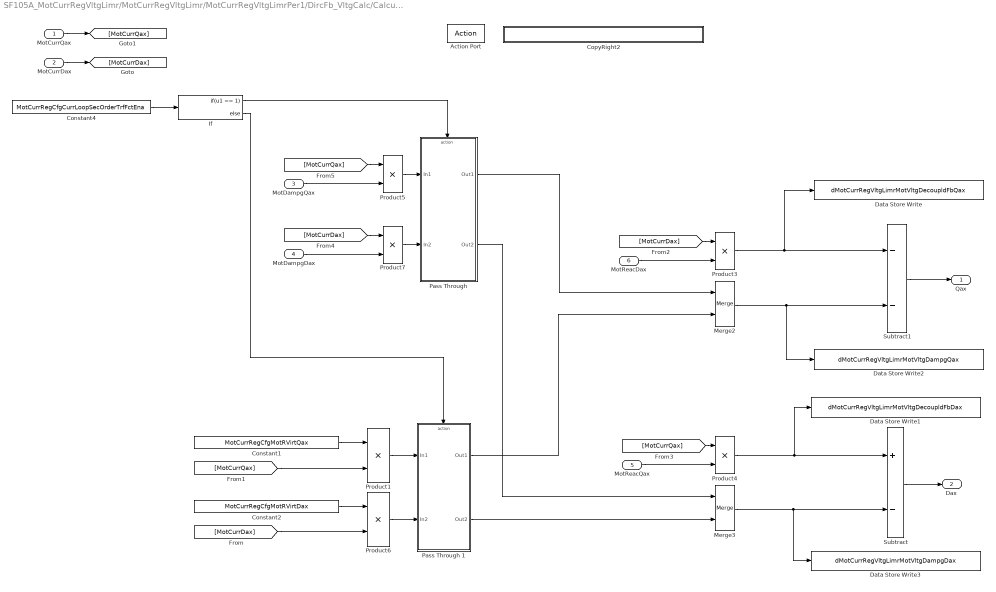
== system SF105A_MotCurrRegVltgLimr/MotCurrRegVltgLimr/MotCurrRegVltgLimrPer1/DircFb_VltgCalc/Calculate Direct Feedback ==
  MotCurrQax : Inport
  MotCurrDax : Inport  Port=2
  MotDampgQax : Inport  RequirementInfo="{'linktype_rmi_doors' '0000bb44 (/E-STEER Core/SubSystem Specifications/Application Functions/SF99/SF105A Current Regulator and Voltage Limiter)' '#SF105A_95' 'true' 'REQ:  SF105A_95' '' } %GIDa_3401c7b5_a1f5_4523_9ada_68582b84022c"  Port=3
  MotDampgDax : Inport  RequirementInfo="{'linktype_rmi_doors' '0000bb44 (/E-STEER Core/SubSystem Specifications/Application Functions/SF99/SF105A Current Regulator and Voltage Limiter)' '#SF105A_95' 'true' 'REQ:  SF105A_95' '' } %GIDa_21977cee_2bd2_49f8_8307_47cf0cbe7c02"  Port=4
  MotReacQax : Inport  RequirementInfo="{'linktype_rmi_doors' '0000bb44 (/E-STEER Core/SubSystem Specifications/Application Functions/SF99/SF105A Current Regulator and Voltage Limiter)' '#SF105A_90' 'true' 'REQ:  SF105A_90' '' } %GIDa_8a4c99a4_fca4_4cf5_ae0f_86bc6ca1febf"  Port=5
  MotReacDax : Inport  RequirementInfo="{'linktype_rmi_doors' '0000bb44 (/E-STEER Core/SubSystem Specifications/Application Functions/SF99/SF105A Current Regulator and Voltage Limiter)' '#SF105A_90' 'true' 'REQ:  SF105A_90' '' } %GIDa_170d645f_2e49_4a68_b0ff_6acc83d1981c"  Port=6
  Action Port : ActionPort  ActionType=else
  Constant1 : Constant  RequirementInfo="{'linktype_rmi_doors' '0000bb44 (/E-STEER Core/SubSystem Specifications/Application Functions/SF99/SF105A Current Regulator and Voltage Limiter)' '#SF105A_93' 'true' 'REQ:  SF105A_93' '' ; 'linktype_rmi_doors' '0000bb44 (/E-STEER Core/SubSystem Specifications/Application Functions/SF99/SF105A Current Regulator and Voltage Limiter)' '#SF105A_96' 'true' 'REQ:  SF105A_96' '' } %GIDa_307e2cf8_46ef_4fd2_bf47_2f1d84b42a20"  Value=MotCurrRegCfgMotRVirtQax
  Constant2 : Constant  RequirementInfo="{'linktype_rmi_doors' '0000bb44 (/E-STEER Core/SubSystem Specifications/Application Functions/SF99/SF105A Current Regulator and Voltage Limiter)' '#SF105A_93' 'true' 'REQ:  SF105A_93' '' ; 'linktype_rmi_doors' '0000bb44 (/E-STEER Core/SubSystem Specifications/Application Functions/SF99/SF105A Current Regulator and Voltage Limiter)' '#SF105A_96' 'true' 'REQ:  SF105A_96' '' } %GIDa_ca61f08e_bc3c_484b_8953_c77aa6be7c4a"  Value=MotCurrRegCfgMotRVirtDax
  Constant4 : Constant  RequirementInfo="{'linktype_rmi_doors' '0000bb44 (/E-STEER Core/SubSystem Specifications/Application Functions/SF99/SF105A Current Regulator and Voltage Limiter)' '#SF105A_95' 'true' 'REQ:  SF105A_95' '' } %GIDa_3bd1aaef_9bee_4467_8a70_f7911309372e"  Value=MotCurrRegCfgCurrLoopSecOrderTrfFctEna
  CopyRight2 : Subsystem  Description=|  mask(Copyright Information){none=on}
      | Copyright info block.                                               
      |                                                                     
      | Place copyright information at the top of every subsystem in design.
      mask prompts: none "No parameters"
      mask help: Place copyright information at the top of every subsystem in design.
      mask Display:
      | NxtrConf = 'Nexteer Confidential';
      | 
      | sys = bdroot; %handle for the current model ("system")
      | first = get_param(sys,'Created');
      | if(isempty(first))
      |     first = datestr(now,'yyyy');
      | else
      |     first = first(end-3:end);  %year is last four digits
      | end
      | 
      | last = get_param(sys,'LastModifiedDate');
      | if isempty(last)
      |     last = datestr(now,'yyyy');
      | else
      |     last = last(end-3:end);
      | end
      | 
      | if strcmp(first,last)
      |     fprintf('%s -- Copyright %s Nexteer',NxtrConf,first)
      | else
      |     fprintf('%s -- %s%s- %s Nexteer',NxtrConf,char(169),first,last)
      | end
  Data Store Write : DataStoreWrite  DataStoreName=dMotCurrRegVltgLimrMotVltgDecoupldFbQax
  Data Store Write1 : DataStoreWrite  DataStoreName=dMotCurrRegVltgLimrMotVltgDecoupldFbDax
  Data Store Write2 : DataStoreWrite  DataStoreName=dMotCurrRegVltgLimrMotVltgDampgQax
  Data Store Write3 : DataStoreWrite  DataStoreName=dMotCurrRegVltgLimrMotVltgDampgDax
  If : If  RequirementInfo="{'linktype_rmi_doors' '0000bb44 (/E-STEER Core/SubSystem Specifications/Application Functions/SF99/SF105A Current Regulator and Voltage Limiter)' '#SF105A_95' 'true' 'REQ:  SF105A_95' '' } %GIDa_4e1c0e54_5425_42bc_a247_78607179434f"  IfExpression=u1 == 1
  Merge2 : Merge  RequirementInfo="{'linktype_rmi_doors' '0000bb44 (/E-STEER Core/SubSystem Specifications/Application Functions/SF99/SF105A Current Regulator and Voltage Limiter)' '#SF105A_95' 'true' 'REQ:  SF105A_95' '' ; 'linktype_rmi_doors' '0000bb44 (/E-STEER Core/SubSystem Specifications/Application Functions/SF99/SF105A Current Regulator and Voltage Limiter)' '#SF105A_96' 'true' 'REQ:  SF105A_96' '' ; 'linktype_rmi_doors' '0000bb44 (/E-STEER Core/SubSystem Specifications/Application Functions/SF99/SF105A Current Regulator and Voltage Limiter)' '#SF105A_97' 'true' 'REQ:  SF105A_97' '' } %GIDa_94d51eec_80e4_4e94_a264_8960fdbac031"
  Merge3 : Merge  RequirementInfo="{'linktype_rmi_doors' '0000bb44 (/E-STEER Core/SubSystem Specifications/Application Functions/SF99/SF105A Current Regulator and Voltage Limiter)' '#SF105A_95' 'true' 'REQ:  SF105A_95' '' ; 'linktype_rmi_doors' '0000bb44 (/E-STEER Core/SubSystem Specifications/Application Functions/SF99/SF105A Current Regulator and Voltage Limiter)' '#SF105A_96' 'true' 'REQ:  SF105A_96' '' ; 'linktype_rmi_doors' '0000bb44 (/E-STEER Core/SubSystem Specifications/Application Functions/SF99/SF105A Current Regulator and Voltage Limiter)' '#SF105A_97' 'true' 'REQ:  SF105A_97' '' } %GIDa_3c43c228_898d_407a_bf34_1f2e98fdef6f"
  Pass Through : Subsystem  RequirementInfo="{'linktype_rmi_doors' '0000bb44 (/E-STEER Core/SubSystem Specifications/Application Functions/SF99/SF105A Current Regulator and Voltage Limiter)' '#SF105A_95' 'true' 'REQ:  SF105A_95' '' } %GIDa_9be2bac2_de64_415e_b5a2_3dcbaafc4b6e"  TreatAsAtomicUnit=on
  Pass Through 1 : Subsystem  RequirementInfo="{'linktype_rmi_doors' '0000bb44 (/E-STEER Core/SubSystem Specifications/Application Functions/SF99/SF105A Current Regulator and Voltage Limiter)' '#SF105A_96' 'true' 'REQ:  SF105A_96' '' } %GIDa_87c347ca_37ba_4bff_a0f3_810118d831db"  TreatAsAtomicUnit=on
  Product1 : Product  RequirementInfo="{'linktype_rmi_doors' '0000bb44 (/E-STEER Core/SubSystem Specifications/Application Functions/SF99/SF105A Current Regulator and Voltage Limiter)' '#SF105A_96' 'true' 'REQ:  SF105A_96' '' } %GIDa_b27c0936_2e09_4b2f_a672_1d05ae2bb0f4"  RndMeth=Zero
  Product3 : Product  RequirementInfo="{'linktype_rmi_doors' '0000bb44 (/E-STEER Core/SubSystem Specifications/Application Functions/SF99/SF105A Current Regulator and Voltage Limiter)' '#SF105A_90' 'true' 'REQ:  SF105A_90' '' ; 'linktype_rmi_doors' '0000bb44 (/E-STEER Core/SubSystem Specifications/Application Functions/SF99/SF105A Current Regulator and Voltage Limiter)' '#SF105A_97' 'true' 'REQ:  SF105A_97' '' } %GIDa_5c2cf5d6_5072_406c_9258_c3956a4ab679"  RndMeth=Zero
  Product4 : Product  RequirementInfo="{'linktype_rmi_doors' '0000bb44 (/E-STEER Core/SubSystem Specifications/Application Functions/SF99/SF105A Current Regulator and Voltage Limiter)' '#SF105A_90' 'true' 'REQ:  SF105A_90' '' ; 'linktype_rmi_doors' '0000bb44 (/E-STEER Core/SubSystem Specifications/Application Functions/SF99/SF105A Current Regulator and Voltage Limiter)' '#SF105A_97' 'true' 'REQ:  SF105A_97' '' } %GIDa_a67fea8e_a6f0_4e04_946b_50b8df6bb922"  RndMeth=Zero
  Product5 : Product  RequirementInfo="{'linktype_rmi_doors' '0000bb44 (/E-STEER Core/SubSystem Specifications/Application Functions/SF99/SF105A Current Regulator and Voltage Limiter)' '#SF105A_95' 'true' 'REQ:  SF105A_95' '' } %GIDa_02d9bf62_4208_4308_9674_ee1c6762fb75"  RndMeth=Zero
  Product6 : Product  RequirementInfo="{'linktype_rmi_doors' '0000bb44 (/E-STEER Core/SubSystem Specifications/Application Functions/SF99/SF105A Current Regulator and Voltage Limiter)' '#SF105A_96' 'true' 'REQ:  SF105A_96' '' } %GIDa_7459c337_d519_4887_b5f7_de6c8da97914"  RndMeth=Zero
  Product7 : Product  RequirementInfo="{'linktype_rmi_doors' '0000bb44 (/E-STEER Core/SubSystem Specifications/Application Functions/SF99/SF105A Current Regulator and Voltage Limiter)' '#SF105A_95' 'true' 'REQ:  SF105A_95' '' } %GIDa_a3ad041c_2fc3_478f_be39_6f0b099c2aac"  RndMeth=Zero
  Subtract : Sum  RequirementInfo="{'linktype_rmi_doors' '0000bb44 (/E-STEER Core/SubSystem Specifications/Application Functions/SF99/SF105A Current Regulator and Voltage Limiter)' '#SF105A_97' 'true' 'REQ:  SF105A_97' '' } %GIDa_1c25cde5_438d_432a_82cf_9eefa44b31de"  Inputs=+-
  Subtract1 : Sum  RequirementInfo="{'linktype_rmi_doors' '0000bb44 (/E-STEER Core/SubSystem Specifications/Application Functions/SF99/SF105A Current Regulator and Voltage Limiter)' '#SF105A_97' 'true' 'REQ:  SF105A_97' '' } %GIDa_37367d35_6b35_4453_8b7a_731b36563e64"  Inputs=--
  Qax : Outport  RequirementInfo="{'linktype_rmi_doors' '0000bb44 (/E-STEER Core/SubSystem Specifications/Application Functions/SF99/SF105A Current Regulator and Voltage Limiter)' '#SF105A_97' 'true' 'REQ:  SF105A_97' '' } %GIDa_c919a0b8_a330_4099_9efc_977fe1aaa1a6"
  Dax : Outport  RequirementInfo="{'linktype_rmi_doors' '0000bb44 (/E-STEER Core/SubSystem Specifications/Application Functions/SF99/SF105A Current Regulator and Voltage Limiter)' '#SF105A_97' 'true' 'REQ:  SF105A_97' '' } %GIDa_1f614ee8_70c9_4e70_90b6_65bbc200af03"  Port=2
  wires:
  Constant2/1 -> Product6/1
  Constant1/1 -> Product1/1
  [MotCurrDax] -> Product6/2
  [MotCurrQax] -> Product1/2
  MotDampgDax/1 -> Product7/2
  [MotCurrDax] -> Product3/1
  MotReacDax/1 -> Product3/2
  [MotCurrQax] -> Product4/1
  MotReacQax/1 -> Product4/2
  Constant4/1 -> If/1
  If/1 -> Pass Through/Action
  If/2 -> Pass Through 1/Action
  [MotCurrDax] -> Product7/1
  [MotCurrQax] -> Product5/1
  MotDampgQax/1 -> Product5/2
  Subtract1/1 -> Qax/1
  Subtract/1 -> Dax/1
  Product7/1 -> Pass Through/2(In2)
  Product5/1 -> Pass Through/1(In1)
  Product1/1 -> Pass Through 1/1(In1)
  Product6/1 -> Pass Through 1/2(In2)
  Product3/1 -> Data Store Write/1, Subtract1/1
  Product4/1 -> Data Store Write1/1, Subtract/1
  Merge2/1 -> Data Store Write2/1, Subtract1/2
  Merge3/1 -> Data Store Write3/1, Subtract/2
  Pass Through 1/1(Out1) -> Merge2/2
  Pass Through/1(Out1) -> Merge2/1
  Pass Through/2(Out2) -> Merge3/1
  Pass Through 1/2(Out2) -> Merge3/2
  MotCurrDax/1 -> [MotCurrDax]
  MotCurrQax/1 -> [MotCurrQax]

== system SF105A_MotCurrRegVltgLimr/MotCurrRegVltgLimr/MotCurrRegVltgLimrPer1/DircFb_VltgCalc/CopyRight2 ==

== system SF105A_MotCurrRegVltgLimr/MotCurrRegVltgLimr/MotCurrRegVltgLimrPer1/DircFb_VltgCalc/Zero Direct Feedback ==
  In1 : Inport
  Action Port : ActionPort  ActionType=then
  Constant{,1..3} (4 alike) : Constant  Value=0  OutDataTypeStr=single
  CopyRight2 : Subsystem  Description=|  mask(Copyright Information){none=on}
      | Copyright info block.                                               
      |                                                                     
      | Place copyright information at the top of every subsystem in design.
      mask prompts: none "No parameters"
      mask help: Place copyright information at the top of every subsystem in design.
      mask Display:
      | NxtrConf = 'Nexteer Confidential';
      | 
      | sys = bdroot; %handle for the current model ("system")
      | first = get_param(sys,'Created');
      | if(isempty(first))
      |     first = datestr(now,'yyyy');
      | else
      |     first = first(end-3:end);  %year is last four digits
      | end
      | 
      | last = get_param(sys,'LastModifiedDate');
      | if isempty(last)
      |     last = datestr(now,'yyyy');
      | else
      |     last = last(end-3:end);
      | end
      | 
      | if strcmp(first,last)
      |     fprintf('%s -- Copyright %s Nexteer',NxtrConf,first)
      | else
      |     fprintf('%s -- %s%s- %s Nexteer',NxtrConf,char(169),first,last)
      | end
  Data Store Write : DataStoreWrite  DataStoreName=dMotCurrRegVltgLimrMotVltgDecoupldFbQax
  Data Store Write1 : DataStoreWrite  DataStoreName=dMotCurrRegVltgLimrMotVltgDecoupldFbDax
  Data Store Write2 : DataStoreWrite  DataStoreName=dMotCurrRegVltgLimrMotVltgDampgQax
  Data Store Write3 : DataStoreWrite  DataStoreName=dMotCurrRegVltgLimrMotVltgDampgDax
  Signal Conversion : SignalConversion
  Signal Conversion1 : SignalConversion
  Qax : Outport
  Dax : Outport  Port=2
  wires:
  In1/1 -> Signal Conversion1/1, Signal Conversion/1
  Signal Conversion/1 -> Qax/1
  Signal Conversion1/1 -> Dax/1
  Constant/1 -> Data Store Write/1
  Constant1/1 -> Data Store Write2/1
  Constant2/1 -> Data Store Write1/1
  Constant3/1 -> Data Store Write3/1

== system SF105A_MotCurrRegVltgLimr/MotCurrRegVltgLimr/MotCurrRegVltgLimrPer1/Kp_Ki_Ctrl_Dax/CopyRight2 ==

== system SF105A_MotCurrRegVltgLimr/MotCurrRegVltgLimr/MotCurrRegVltgLimrPer1/Kp_Ki_Ctrl_Dax/If Action Subsystem ==
  In1 : Inport
  Action Port : ActionPort  ActionType=then
  CopyRight2 : Subsystem  Description=|  mask(Copyright Information){none=on}
      | Copyright info block.                                               
      |                                                                     
      | Place copyright information at the top of every subsystem in design.
      mask prompts: none "No parameters"
      mask help: Place copyright information at the top of every subsystem in design.
      mask Display:
      | NxtrConf = 'Nexteer Confidential';
      | 
      | sys = bdroot; %handle for the current model ("system")
      | first = get_param(sys,'Created');
      | if(isempty(first))
      |     first = datestr(now,'yyyy');
      | else
      |     first = first(end-3:end);  %year is last four digits
      | end
      | 
      | last = get_param(sys,'LastModifiedDate');
      | if isempty(last)
      |     last = datestr(now,'yyyy');
      | else
      |     last = last(end-3:end);
      | end
      | 
      | if strcmp(first,last)
      |     fprintf('%s -- Copyright %s Nexteer',NxtrConf,first)
      | else
      |     fprintf('%s -- %s%s- %s Nexteer',NxtrConf,char(169),first,last)
      | end
  Out1 : Outport
  wires:
  In1/1 -> Out1/1

== system SF105A_MotCurrRegVltgLimr/MotCurrRegVltgLimr/MotCurrRegVltgLimrPer1/Kp_Ki_Ctrl_Dax/If Action Subsystem1 ==
  In1 : Inport
  Action Port : ActionPort  ActionType=else
  CopyRight2 : Subsystem  Description=|  mask(Copyright Information){none=on}
      | Copyright info block.                                               
      |                                                                     
      | Place copyright information at the top of every subsystem in design.
      mask prompts: none "No parameters"
      mask help: Place copyright information at the top of every subsystem in design.
      mask Display:
      | NxtrConf = 'Nexteer Confidential';
      | 
      | sys = bdroot; %handle for the current model ("system")
      | first = get_param(sys,'Created');
      | if(isempty(first))
      |     first = datestr(now,'yyyy');
      | else
      |     first = first(end-3:end);  %year is last four digits
      | end
      | 
      | last = get_param(sys,'LastModifiedDate');
      | if isempty(last)
      |     last = datestr(now,'yyyy');
      | else
      |     last = last(end-3:end);
      | end
      | 
      | if strcmp(first,last)
      |     fprintf('%s -- Copyright %s Nexteer',NxtrConf,first)
      | else
      |     fprintf('%s -- %s%s- %s Nexteer',NxtrConf,char(169),first,last)
      | end
  Out1 : Outport
  wires:
  In1/1 -> Out1/1

== system SF105A_MotCurrRegVltgLimr/MotCurrRegVltgLimr/MotCurrRegVltgLimrPer1/Kp_Ki_Ctrl_Qax/CopyRight2 ==
